simulink model "Kin_v_BHA_cc"  (R2018b)
settings: Solver=FixedStepDiscrete  StartTime=0.0  StopTime=10  FixedStep=0.010  RelTol=1e-3  EnableMultiTasking=on
PostLoadFcn:
  | , if any(exist('dsrtsu_mdlpostloadfcn', 'file') == [2, 3, 6]), try dsrtsu_mdlpostloadfcn('Execute', bdroot); catch fprintf('Error in PostLoadFcn (dsrtsu_mdlpostloadfcn) for model "%s":\n %s\n', bdroot, lasterr); end, end,
undefined symbols (not defined in the file or in its folder): DiscIntNeverNeededParam, lData
libraries: libo_robotics x1
settings Model: DSRTSU_INTERNAL_RTI_VER=440  DSRTSU_INTERNAL_RTI_TYPE=rti1007  DSRTSU_INTERNAL_RTIFPGA=30  Creator=Mahl  LastModifiedBy=Müller
settings DataIOCC: LimitDataPoints=on  SaveFormat=Array
settings OptimizationCC: BlockReduction=off  OptimizeBlockIOStorage=off  BufferReuse=off  GlobalBufferReuse=off  ExpressionFolding=off  ExpressionDepthLimit=2147483647  LocalBlockOutputs=off  LifeSpan=inf  OptimizeDataStoreBuffers=off  BusAssignmentInplaceUpdate=off
settings DebuggingCC: SolverPrmCheckMsg=warning  AllowSymbolicDim=off  StateNameClashWarn=warning  SFUnexpectedBacktrackingDiag=warning  SFNoUnconditionalDefaultTransitionDiag=warning  SFExecutionAtInitializationDiag=none
settings HardwareCC: ProdBitPerPointer=32  ProdBitPerSizeT=32  ProdBitPerPtrDiffT=32  ProdLargestAtomicFloat=None  ProdEndianess=BigEndian  ProdWordSize=32  ProdHWDeviceType=Generic->Custom  TargetIntDivRoundTo=Zero  TargetEndianess=BigEndian  TargetHWDeviceType=Generic->Custom
settings ModelReferenceCC: PropagateSignalLabelsOutOfModel=off
settings SFSimCC: SimUseLocalCustomCode=off
settings RTWCC: SystemTargetFile=rti1103.tlc  MakeCommand=make_rti  TemplateMakefile=rti1103.tmf  Description=dSPACE DS1103 Hardware Platform  RTWUseLocalCustomCode=off
settings CodeAppCC: StateflowObjectComments=on
settings STFCustomTargetCC: ParMdlRefBuildCompliant=on  GeneratePreprocessorConditionals=Disable all  MatFileLogging=on  CPPClassGenCompliant=on  GRTInterface=on  SystemTargetFile=rti1103.tlc
settings GRTTargetCC: TargetLangStandard=C89/C90 (ANSI)  CompOptLevelCompliant=off  ConcurrentExecutionCompliant=off  GeneratePreprocessorConditionals=Disable all  CombineOutputUpdateFcns=off  GRTInterface=on  UseToolchainInfoCompliant=off  ExtModeMexFile=noextcomm
settings ConfigComp: CovMetricSettings=dw  CovHtmlReporting=on  CovSaveCumulativeToWorkspaceVar=on  CovSaveSingleToWorkspaceVar=on  CovExternalEMLEnable=off

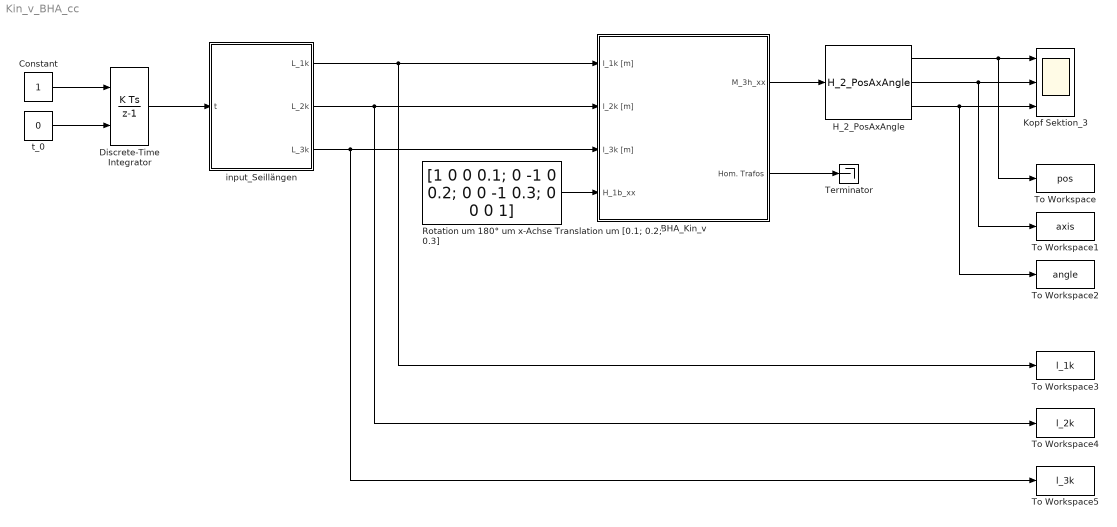
== system Kin_v_BHA_cc ==
  BHA_Kin_v : Subsystem
  Constant : Constant
  Discrete-Time Integrator : DiscreteIntegrator  InitialConditionSource=external  SampleTime=0.010  ICPrevOutput=DiscIntNeverNeededParam  ICPrevScaledInput=DiscIntNeverNeededParam
  H_2_PosAxAngle : libo_robotics/Kinematics/H_2_PosAxAngle  SystemSampleTime=-1
  Kopf Sektion_3 : Scope  NumInputPorts=3
  Rotation um 180° um x-Achse Translation um [0.1; 0.2; 0.3] : Constant  Value=[1 0 0 0.1; 0 -1 0 0.2; 0 0 -1 0.3; 0 0 0 1]
  Terminator : Terminator
  To Workspace : ToWorkspace  VariableName=pos  SaveFormat=Structure With Time  SampleTime=-1
      settings: Decimation=10
  To Workspace1 : ToWorkspace  VariableName=axis  SaveFormat=Structure With Time  SampleTime=-1
      settings: Decimation=10
  To Workspace2 : ToWorkspace  VariableName=angle  SaveFormat=Structure With Time  SampleTime=-1
      settings: Decimation=10
  To Workspace3 : ToWorkspace  VariableName=l_1k  SaveFormat=Structure With Time  SampleTime=-1
      settings: Decimation=10
  To Workspace4 : ToWorkspace  VariableName=l_2k  SaveFormat=Structure With Time  SampleTime=-1
      settings: Decimation=10
  To Workspace5 : ToWorkspace  VariableName=l_3k  SaveFormat=Structure With Time  SampleTime=-1
      settings: Decimation=10
  input_Seillängen : Subsystem
  t_0 : Constant  Value=0
  wires:
  Discrete-Time Integrator/1 -> input_Seillängen/1(t)
  Constant/1 -> Discrete-Time Integrator/1
  t_0/1 -> Discrete-Time Integrator/2
  H_2_PosAxAngle/1 -> Kopf Sektion_3/1, To Workspace/1
  H_2_PosAxAngle/2 -> Kopf Sektion_3/2, To Workspace1/1
  H_2_PosAxAngle/3 -> Kopf Sektion_3/3, To Workspace2/1
  input_Seillängen/1(L_1k) -> BHA_Kin_v/1(l_1k [m]), To Workspace3/1
  input_Seillängen/3(L_3k) -> BHA_Kin_v/3(l_3k [m]), To Workspace5/1
  BHA_Kin_v/1("M_3h_xx ") -> H_2_PosAxAngle/1
  BHA_Kin_v/2(Hom. Trafos) -> Terminator/1
  Rotation um 180° um x-Achse Translation um [0.1; 0.2; 0.3]/1 -> BHA_Kin_v/4(H_1b_xx)
  input_Seillängen/2(L_2k) -> BHA_Kin_v/2(l_2k [m]), To Workspace4/1

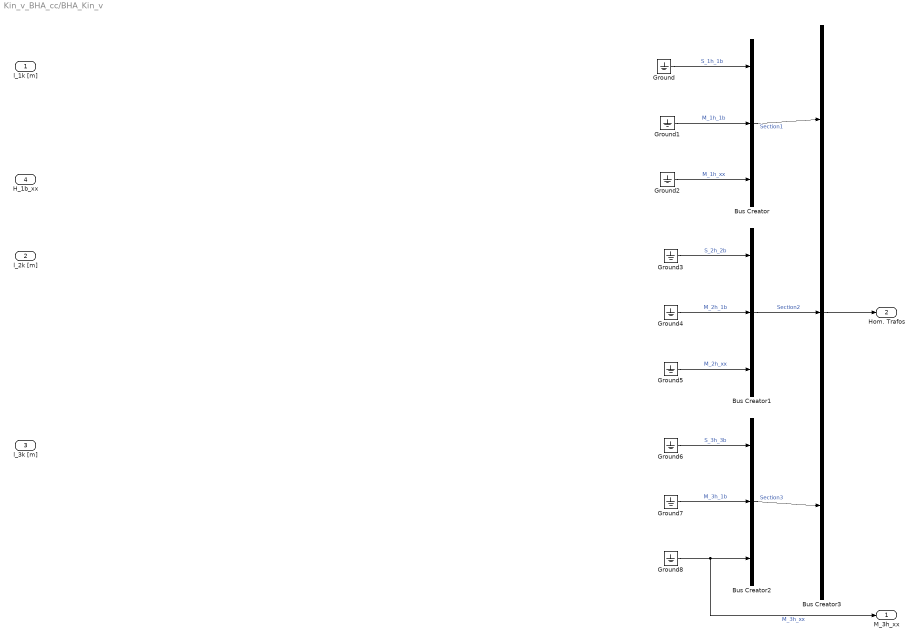
== system Kin_v_BHA_cc/BHA_Kin_v ==
  l_1k [m] : Inport
  l_2k [m] : Inport  Port=2
  l_3k [m] : Inport  Port=3
  H_1b_xx : Inport  Port=4
  Bus Creator{,1..3} (4 alike) : BusCreator  Inputs=3
  Ground{,1..8} (9 alike) : Ground
  "M_3h_xx " : Outport
  Hom. Trafos : Outport  Port=2
  wires:
  Ground1/1 -> Bus Creator/2  "M_1h_1b"
  Ground2/1 -> Bus Creator/3  "M_1h_xx"
  Ground/1 -> Bus Creator/1  "S_1h_1b"
  Ground3/1 -> Bus Creator1/1  "S_2h_2b"
  Ground4/1 -> Bus Creator1/2  "M_2h_1b"
  Ground5/1 -> Bus Creator1/3  "M_2h_xx"
  Ground7/1 -> Bus Creator2/2  "M_3h_1b"
  Ground8/1 -> Bus Creator2/3, "M_3h_xx "/1  "M_3h_xx"
  Ground6/1 -> Bus Creator2/1  "S_3h_3b"
  Bus Creator/1 -> Bus Creator3/1  "Section1"
  Bus Creator1/1 -> Bus Creator3/2  "Section2"
  Bus Creator2/1 -> Bus Creator3/3  "Section3"
  Bus Creator3/1 -> Hom. Trafos/1

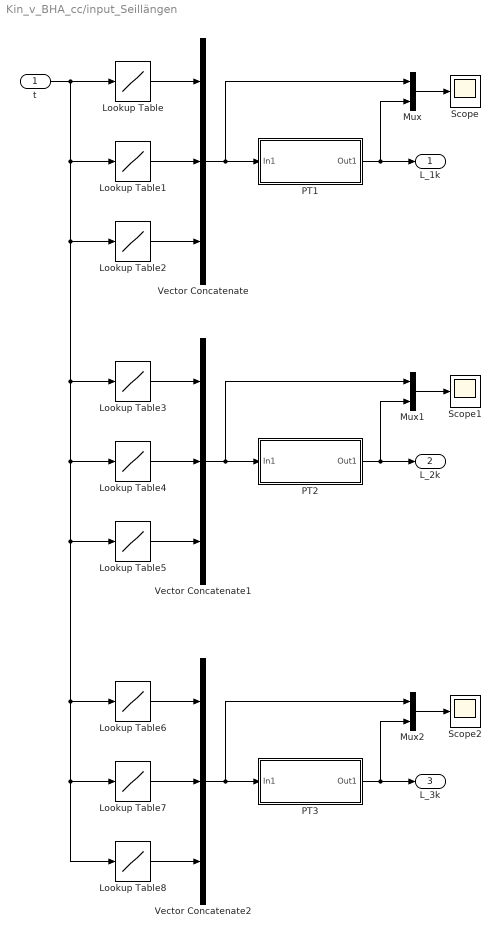
== system Kin_v_BHA_cc/input_Seillängen ==
  t : Inport
  Lookup Table : Lookup_n-D  NumberOfTableDimensions=1  BreakpointsForDimension1=lData.time  Table=lData.l_1k(1,:)  InterpMethod=Nearest  ExtrapMethod=Clip  InternalRulePriority=Speed  InputSameDT=on
      settings: AttributesFormatString=%<Table>
  Lookup Table1 : Lookup_n-D  NumberOfTableDimensions=1  BreakpointsForDimension1=lData.time  Table=lData.l_1k(2,:)  InterpMethod=Nearest  ExtrapMethod=Clip  InternalRulePriority=Speed  InputSameDT=on
      settings: AttributesFormatString=%<Table>
  Lookup Table2 : Lookup_n-D  NumberOfTableDimensions=1  BreakpointsForDimension1=lData.time  Table=lData.l_1k(3,:)  InterpMethod=Nearest  ExtrapMethod=Clip  InternalRulePriority=Speed  InputSameDT=on
      settings: AttributesFormatString=%<Table>
  Lookup Table3 : Lookup_n-D  NumberOfTableDimensions=1  BreakpointsForDimension1=lData.time  Table=lData.l_2k(1,:)  InterpMethod=Nearest  ExtrapMethod=Clip  InternalRulePriority=Speed  InputSameDT=on
      settings: AttributesFormatString=%<Table>
  Lookup Table4 : Lookup_n-D  NumberOfTableDimensions=1  BreakpointsForDimension1=lData.time  Table=lData.l_2k(2,:)  InterpMethod=Nearest  ExtrapMethod=Clip  InternalRulePriority=Speed  InputSameDT=on
      settings: AttributesFormatString=%<Table>
  Lookup Table5 : Lookup_n-D  NumberOfTableDimensions=1  BreakpointsForDimension1=lData.time  Table=lData.l_2k(3,:)  InterpMethod=Nearest  ExtrapMethod=Clip  InternalRulePriority=Speed  InputSameDT=on
      settings: AttributesFormatString=%<Table>
  Lookup Table6 : Lookup_n-D  NumberOfTableDimensions=1  BreakpointsForDimension1=lData.time  Table=lData.l_3k(1,:)  InterpMethod=Nearest  ExtrapMethod=Clip  InternalRulePriority=Speed  InputSameDT=on
      settings: AttributesFormatString=%<Table>
  Lookup Table7 : Lookup_n-D  NumberOfTableDimensions=1  BreakpointsForDimension1=lData.time  Table=lData.l_3k(2,:)  InterpMethod=Nearest  ExtrapMethod=Clip  InternalRulePriority=Speed  InputSameDT=on
      settings: AttributesFormatString=%<Table>
  Lookup Table8 : Lookup_n-D  NumberOfTableDimensions=1  BreakpointsForDimension1=lData.time  Table=lData.l_3k(3,:)  InterpMethod=Nearest  ExtrapMethod=Clip  InternalRulePriority=Speed  InputSameDT=on
      settings: AttributesFormatString=%<Table>
  Mux : Mux  Inputs=2
  Mux1 : Mux  Inputs=2
  Mux2 : Mux  Inputs=2
  PT1 : Subsystem
  PT2 : Subsystem
  PT3 : Subsystem
  Scope : Scope
  Scope1 : Scope
  Scope2 : Scope
  Vector Concatenate : Concatenate  NumInputs=3  Mode=Multidimensional array
  Vector Concatenate1 : Concatenate  NumInputs=3  Mode=Multidimensional array
  Vector Concatenate2 : Concatenate  NumInputs=3  Mode=Multidimensional array
  L_1k : Outport
  L_2k : Outport  Port=2
  L_3k : Outport  Port=3
  wires:
  t/1 -> Lookup Table1/1, Lookup Table2/1, Lookup Table3/1, Lookup Table4/1, Lookup Table5/1, Lookup Table6/1, Lookup Table7/1, Lookup Table8/1, Lookup Table/1
  Lookup Table/1 -> Vector Concatenate/1
  Lookup Table1/1 -> Vector Concatenate/2
  Lookup Table2/1 -> Vector Concatenate/3
  Vector Concatenate/1 -> PT1/1(In1), Mux/1
  PT1/1(Out1) -> L_1k/1, Mux/2
  Mux/1 -> Scope/1
  Lookup Table3/1 -> Vector Concatenate1/1
  Lookup Table4/1 -> Vector Concatenate1/2
  Lookup Table5/1 -> Vector Concatenate1/3
  Vector Concatenate1/1 -> Mux1/1, PT2/1(In1)
  PT2/1(Out1) -> Mux1/2, L_2k/1
  Mux1/1 -> Scope1/1
  Lookup Table6/1 -> Vector Concatenate2/1
  Lookup Table7/1 -> Vector Concatenate2/2
  Lookup Table8/1 -> Vector Concatenate2/3
  Vector Concatenate2/1 -> PT3/1(In1), Mux2/1
  PT3/1(Out1) -> L_3k/1, Mux2/2
  Mux2/1 -> Scope2/1

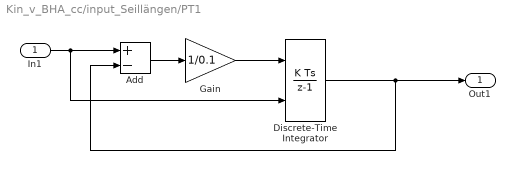
== system Kin_v_BHA_cc/input_Seillängen/PT1 ==
  In1 : Inport
  Add : Sum  Inputs=+-
  Discrete-Time Integrator : DiscreteIntegrator  InitialConditionSource=external  SampleTime=0.010  ICPrevOutput=DiscIntNeverNeededParam  ICPrevScaledInput=DiscIntNeverNeededParam
  Gain : Gain  Gain=1/0.1
  Out1 : Outport
  wires:
  In1/1 -> Add/1, Discrete-Time Integrator/2
  Add/1 -> Gain/1
  Discrete-Time Integrator/1 -> Out1/1, Add/2
  Gain/1 -> Discrete-Time Integrator/1

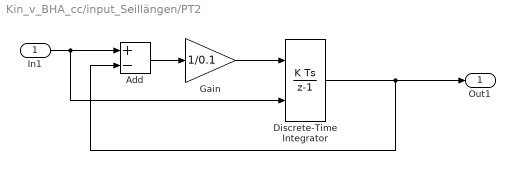
== system Kin_v_BHA_cc/input_Seillängen/PT2 ==
  In1 : Inport
  Add : Sum  Inputs=+-
  Discrete-Time Integrator : DiscreteIntegrator  InitialConditionSource=external  SampleTime=0.010  ICPrevOutput=DiscIntNeverNeededParam  ICPrevScaledInput=DiscIntNeverNeededParam
  Gain : Gain  Gain=1/0.1
  Out1 : Outport
  wires:
  Gain/1 -> Discrete-Time Integrator/1
  Discrete-Time Integrator/1 -> Add/2, Out1/1
  Add/1 -> Gain/1
  In1/1 -> Discrete-Time Integrator/2, Add/1

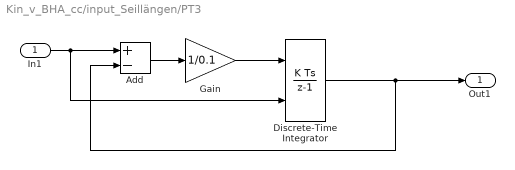
== system Kin_v_BHA_cc/input_Seillängen/PT3 ==
  In1 : Inport
  Add : Sum  Inputs=+-
  Discrete-Time Integrator : DiscreteIntegrator  InitialConditionSource=external  SampleTime=0.010  ICPrevOutput=DiscIntNeverNeededParam  ICPrevScaledInput=DiscIntNeverNeededParam
  Gain : Gain  Gain=1/0.1
  Out1 : Outport
  wires:
  In1/1 -> Add/1, Discrete-Time Integrator/2
  Add/1 -> Gain/1
  Discrete-Time Integrator/1 -> Out1/1, Add/2
  Gain/1 -> Discrete-Time Integrator/1
